simulink subsystem "Final_Project_PreBusUnpack_20260601_105527"  (R2024a)
settings: Solver=VariableStepAuto  StartTime=0.0  StopTime=10.0  RelTol=1e-3
values from neighbouring files (symbols this model uses):
  D = hypot(Ep(:,1)-Tp(:,1)',Ep(:,2)-Tp(:,2)')    [pp_compare_stage.m]    (also in pp_diag_path.m; pp_t09_clear.m = hypot(Ep(:,1)-Tperim(:,1)', Ep(:,2)-Tperim(:,2)'); pp_tune2.m)
undefined symbols (not defined in the file or in its folder): waypoints
libraries: CarMaker4SL x116, simulink x1
(part 1 of 7)
settings Model: Creator=junho.lee  LastModifiedBy=hajin

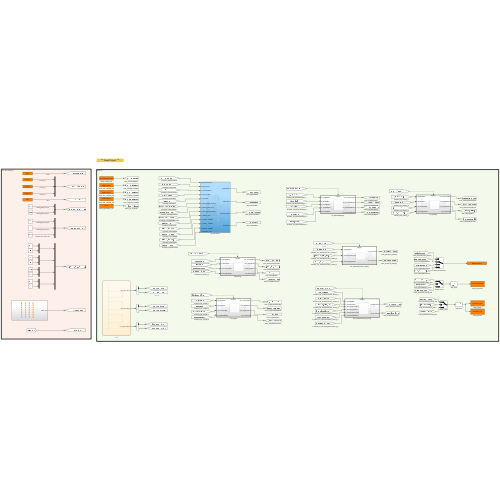
[thumbnail: Simulink's stored preview of the top-level diagram]
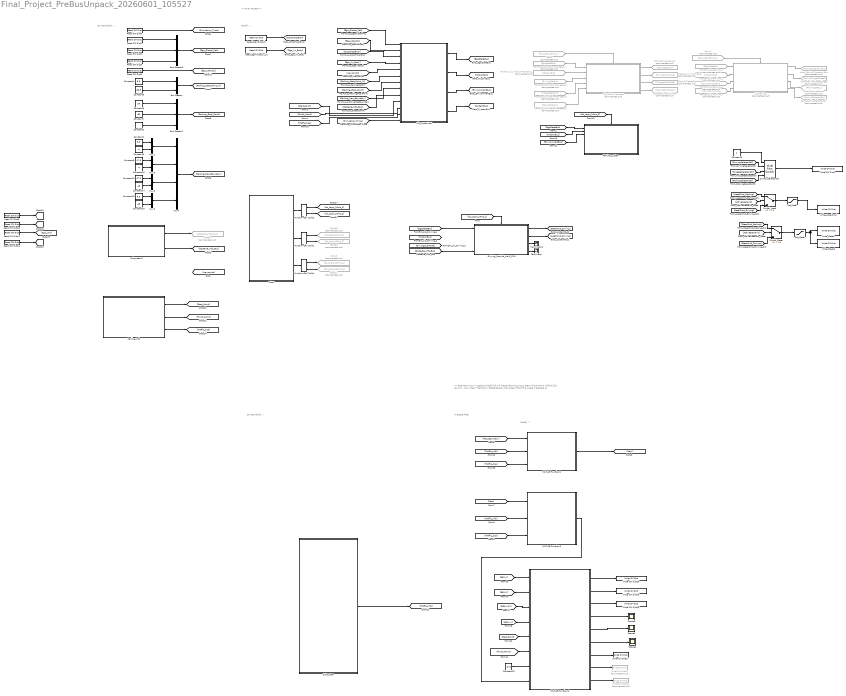
== system Final_Project_PreBusUnpack_20260601_105527 ==
  note: Do Not Modify !!
  note: *** Final Project ***
  note: Modify !!
  note: Do Not Modify !!
  note: Average Filter
  note: *** Path Planning ***
      |
      | Scenario: 장애물 회피 & 주차 Path Planning
      | Input: Start / Finish Point + 선행차량 정보 (Pos X/Y, Yaw, Size) + Collision / Object Sensor Info
      | Output: Front Tire Angle + Desired Ax
  note: Modify !!
  Bus Creator : BusCreator  Inputs=2
  Bus Creator1 : BusCreator  Inputs=3
  Bus Creator3 : BusCreator  Inputs=3
  Chart : Stateflow chart  TreatAsAtomicUnit=on
  Constant1 : Constant  Value=5.5
  Constant10 : Constant  Value=-4
  Constant13 : Constant  Value=47.5
  Constant14 : Constant  Value=-45
  Constant15 : Constant  Value=5.5
  Constant16 : Constant  Value=-45
  Constant2 : Constant  Value=2*pi/3
  Constant23 : Constant  Value=-pi/2
  Constant3 : Constant
  Constant4 : Constant  Value=5.5
  Constant5 : Constant  Value=-36.5
  Constant6 : Constant  Value=35
  Constant7 : Constant  Value=-30
  Constant8 : Constant  Value=47.5
  Constant9 : Constant  Value=-4
  Driving_Module_Ver.3_PSH : Subsystem
  From2 : From  Commented=on  GotoTag=do_Logic_50ms_1
  From5 : From  Commented=on  GotoTag=do_Logic_10ms_1
  FromExt_Lib_MissionManager_1 : From  Commented=on  GotoTag=EgoStateBus
  FromExt_Lib_MissionManager_2 : From  Commented=on  GotoTag=MissionBus
  FromExt_Lib_MissionManager_3 : From  Commented=on  GotoTag=DrivingStatus
  FromExt_Lib_MissionManager_4 : From  Commented=on  GotoTag=TollgateStatus
  FromExt_Lib_MissionManager_5 : From  Commented=on  GotoTag=ParkingStatus
  FromExt_Lib_Parking_1 : From  Commented=on  GotoTag=EgoStateBus
  FromExt_Lib_Parking_2 : From  Commented=on  GotoTag=MissionBus
  FromExt_Lib_Parking_3 : From  Commented=on  GotoTag=EnvironmentBus
  FromExt_Lib_Parking_4 : From  Commented=on  GotoTag=ParkingSubMode
  Function-Call Split1 : FunctionCallSplit  IconShape=distinctive  NumOutputPorts=2  OutputPortLayout=default
  Function-Call Split2 : FunctionCallSplit  IconShape=distinctive  NumOutputPorts=2  OutputPortLayout=default
  Function-Call Split4 : FunctionCallSplit  IconShape=distinctive  NumOutputPorts=2  OutputPortLayout=default
  Goto11 : Goto  Commented=on  GotoTag=do_Logic_100ms_2
  Goto28 : Goto  Commented=on  GotoTag=do_Logic_50ms_1
  Goto3 : Goto  Commented=on  GotoTag=do_Logic_100ms_1
  Goto30 : Goto  Commented=on  GotoTag=do_Logic_50ms_2
  Goto9 : Goto  Commented=on  GotoTag=Obstacle_Info_Mux
  Goto_ActiveScenario : Goto  Commented=on  GotoTag=ActiveScenario
  Goto_DrivingSubMode : Goto  Commented=on  GotoTag=DrivingSubMode
  Goto_ParkingSelectorCtrl : Goto  Commented=on  GotoTag=ParkingSelectorCtrl
  Goto_ParkingStatus : Goto  Commented=on  GotoTag=ParkingStatus
  Goto_ParkingSubMode : Goto  Commented=on  GotoTag=ParkingSubMode
  Goto_ParkingTargetSpeed : Goto  Commented=on  GotoTag=ParkingTargetSpeed
  Goto_ParkingTrajectoryBus : Goto  Commented=on  GotoTag=ParkingTrajectoryBus
  Goto_TollgateSubMode : Goto  Commented=on  GotoTag=TollgateSubMode
  Lib_MissionManager : Subsystem  Commented=on
  Lib_Parking : Subsystem  Commented=on
  Lib_Supervisor : Subsystem
  MATLAB Function2 : MATLAB Function  TreatAsAtomicUnit=on
  MATLAB Function3 : MATLAB Function  TreatAsAtomicUnit=on
  MATLAB Function6 : MATLAB Function  TreatAsAtomicUnit=on
  Mux{2,5,8..9} (4 alike) : Mux  Inputs=2
  Mux4 : Mux
  Parking_Info : Subsystem
  Parking_system : Subsystem
  Read CM Dict1 : CarMaker4SL/Read CM Dict  xname=Car.Fr1.tx  xsync=off  xstime=Inherited
  Read CM Dict10 : CarMaker4SL/Read CM Dict  xname=Car.Fr1.ty  xsync=off  xstime=Continuous
  Read CM Dict11 : CarMaker4SL/Read CM Dict  xname=Car.v  xsync=off  xstime=Continuous
  Read CM Dict12 : CarMaker4SL/Read CM Dict  xname=Car.Fr1.rz  xsync=off  xstime=Continuous
  Read CM Dict2 : CarMaker4SL/Read CM Dict  xname=Car.Fr1.ty  xsync=off  xstime=Inherited
  Read CM Dict3 : CarMaker4SL/Read CM Dict  xname=Car.Fr1.rz  xsync=off  xstime=Inherited
  Read CM Dict4 : CarMaker4SL/Read CM Dict  xname=Time  xsync=off  xstime=Inherited
  Read CM Dict5 : CarMaker4SL/Read CM Dict  xname=Car.v  xsync=off  xstime=Inherited
  Read CM Dict9 : CarMaker4SL/Read CM Dict  xname=Car.Fr1.tx  xsync=off  xstime=Continuous
  Read_DevDist_Lib : CarMaker4SL/Read CM Dict  xname=Car.Road.Path.DevDist  xsync=off  xstime=Inherited
  Read_EgoVxBody_Lib : CarMaker4SL/Read CM Dict  xname=Car.vx  xsync=off  xstime=Inherited
  Sat_Accel : Saturate  UpperLimit=3.0  LowerLimit=-5.0
  Sat_Steer : Saturate  UpperLimit=pi/6  LowerLimit=-pi/6
  Scope1 : Scope
  Scope2 : Scope
  Scope3 : Scope
  Subsystem : Subsystem
  Subsystem1 : Subsystem
  Switch_Accel : Switch  Criteria=u2 > Threshold  Threshold=2.5
  Switch_SelectorCtrl : MultiPortSwitch  DataPortOrder=Specify indices  DataPortIndices={1, 2, 3}  OutDataTypeStr=double
  Switch_Steer : Switch  Criteria=u2 > Threshold  Threshold=2.5
  Terminator : Terminator
  Terminator1 : Terminator
  Write CM Dict14 : CarMaker4SL/Write CM Dict  xname=Car.CFL.rz_ext  xsync=off
  Write CM Dict15 : CarMaker4SL/Write CM Dict  xname=Car.CFR.rz_ext  xsync=off
  Write CM Dict16 : CarMaker4SL/Write CM Dict  Commented=on  xname=VC.Brake  xsync=off
  Write CM Dict17 : CarMaker4SL/Write CM Dict  xname=DM.SelectorCtrl  xsync=off
  Write CM Dict18 : CarMaker4SL/Write CM Dict  Commented=on  xname=VC.Gas  xsync=off
  Write CM Dict19 : CarMaker4SL/Write CM Dict  xname=AccelCtrl.DesiredAx  xsync=off
  Write CM Dict4 : CarMaker4SL/Write CM Dict  xname=DM.SelectorCtrl  xsync=off
  Write_AccelCmd : CarMaker4SL/Write CM Dict  xname=AccelCtrl.DesiredAx  xsync=off
  Write_SteerL : CarMaker4SL/Write CM Dict  xname=Car.CFL.rz_ext  xsync=off
  Write_SteerR : CarMaker4SL/Write CM Dict  xname=Car.CFR.rz_ext  xsync=off
  wires:
  Constant13/1 -> Mux8/1
  Subsystem1/1(Traffic_Info) -> Goto9/1
  Read CM Dict1/1 -> Bus Creator3/1  "Car_Fr1_tx"
  Read CM Dict3/1 -> Bus Creator3/3  "Car_Fr1_rz"
  Constant4/1 -> Bus Creator/1  "Parking_Start_Point_X"
  Chart/2(do_Logic_50ms()) -> Function-Call Split1/1
  Function-Call Split2/1 -> [do_Logic_10ms_1]
  Function-Call Split1/2 -> Goto30/1
  Read CM Dict4/1 -> [Simulation_Time]  "Time"
  Constant9/1 -> Mux2/2
  Bus Creator1/1 -> [Parking_Goal_Point]
  Mux8/1 -> Mux4/3
  Constant6/1 -> Bus Creator1/1  "Parking_Goal_Point_X"
  Constant1/1 -> Mux2/1
  Constant16/1 -> Mux9/2
  Read CM Dict2/1 -> Bus Creator3/2  "Car_Fr1_ty"
  Function-Call Split1/1 -> Goto28/1
  Constant5/1 -> Bus Creator/2  "Parking_Start_Point_Y"
  Chart/1(do_Logic_10ms()) -> Function-Call Split2/1
  Constant7/1 -> Bus Creator1/2  "Parking_Goal_Point_Y"
  Read CM Dict5/1 -> [Ego_Velocity]  "Car.v"
  Constant15/1 -> Mux9/1
  Constant10/1 -> Mux5/2
  Bus Creator3/1 -> [Ego_Global_Pos]
  Constant14/1 -> Mux8/2
  Function-Call Split2/2 -> [do_Logic_10ms_2]
  Bus Creator/1 -> [Parking_Start_Point_XY]
  Mux9/1 -> Mux4/4
  Mux2/1 -> Mux4/1
  Mux4/1 -> [Parking_Map_Boundary]
  Constant8/1 -> Mux5/1
  Constant2/1 -> Bus Creator1/3  "Parking_Goal_Point_Yaw"
  Mux5/1 -> Mux4/2
  Chart/3(do_Logic_100ms()) -> Function-Call Split4/1
  Function-Call Split4/1 -> Goto3/1
  Function-Call Split4/2 -> Goto11/1
  Sat_Steer/1 -> Write_SteerR/1, Write_SteerL/1
  Read_DevDist_Lib/1 -> [CrossTrackError]
  Read_EgoVxBody_Lib/1 -> [Ego_Vx_Body]
  [Ego_Global_Pos] -> Lib_Supervisor/1(In_Ego_Global_Pos)
  [Ego_Velocity] -> Lib_Supervisor/2(In_Ego_Velocity)
  [CrossTrackError] -> Lib_Supervisor/3(In_CrossTrackError)
  [Ego_Vx_Body] -> Lib_Supervisor/4(In_Ego_Vx_Body)
  [waypoints] -> Lib_Supervisor/5(In_Waypoints)
  [Parking_Start_Point_XY] -> Lib_Supervisor/6(In_Parking_Start_Point_XY)
  [Parking_Goal_Point] -> Lib_Supervisor/7(In_Parking_Goal_Point)
  [Parking_Map_Boundary] -> Lib_Supervisor/8(In_Parking_Map_Boundary)
  [Simulation_Time] -> Lib_Supervisor/13(In_Simulation_Time)
  Lib_Supervisor/1(EgoStateBus) -> [EgoStateBus]
  Lib_Supervisor/2(MissionBus) -> [MissionBus]
  Lib_Supervisor/3(EnvironmentBus) -> [EnvironmentBus]
  Lib_Supervisor/4(SystemBus) -> [SystemBus]
  Lib_MissionManager/1(Out_ActiveScenario) -> Goto_ActiveScenario/1
  Lib_MissionManager/2(Out_DrivingSubMode) -> Goto_DrivingSubMode/1
  Lib_MissionManager/3(Out_TollgateSubMode) -> Goto_TollgateSubMode/1
  Lib_MissionManager/4(Out_ParkingSubMode) -> Goto_ParkingSubMode/1
  Lib_Parking/1(Out_TrajectoryBus) -> Goto_ParkingTrajectoryBus/1
  Lib_Parking/2(Out_TargetSpeed) -> Goto_ParkingTargetSpeed/1
  Lib_Parking/3(Out_ParkingStatus) -> Goto_ParkingStatus/1
  FromExt_Lib_MissionManager_1/1 -> Lib_MissionManager/1(In_EgoStateBus)
  FromExt_Lib_MissionManager_2/1 -> Lib_MissionManager/2(In_MissionBus)
  FromExt_Lib_MissionManager_3/1 -> Lib_MissionManager/3(In_DrivingStatus)
  FromExt_Lib_MissionManager_4/1 -> Lib_MissionManager/4(In_TollgateStatus)
  FromExt_Lib_MissionManager_5/1 -> Lib_MissionManager/5(In_ParkingStatus)
  [EgoStateBus] -> Driving_Module_Ver.3_PSH/1(In_EgoStateBus)
  FromExt_Lib_Parking_1/1 -> Lib_Parking/1(In_EgoStateBus)
  FromExt_Lib_Parking_2/1 -> Lib_Parking/2(In_MissionBus)
  FromExt_Lib_Parking_3/1 -> Lib_Parking/3(In_EnvironmentBus)
  FromExt_Lib_Parking_4/1 -> Lib_Parking/4(In_ParkingSubMode)
  From5/1 -> Lib_MissionManager/Trigger
  [do_Logic_10ms_1] -> Driving_Module_Ver.3_PSH/Trigger
  From2/1 -> Lib_Parking/Trigger
  [SteerCmd_Parking] -> Switch_Steer/1
  [ActiveScenario] -> Switch_Steer/2
  [SteerCmd_Driving] -> Switch_Steer/3
  Switch_Steer/1 -> Sat_Steer/1
  [AccelCmd_Parking] -> Switch_Accel/1
  [ActiveScenario] -> Switch_Accel/2
  [AccelCmd_Driving] -> Switch_Accel/3
  Switch_Accel/1 -> Sat_Accel/1
  Lib_Parking/4(Out_SelectorCtrl) -> Goto_ParkingSelectorCtrl/1
  [DrivingSelectorCtrl] -> Switch_SelectorCtrl/2
  [TollgateSelectorCtrl] -> Switch_SelectorCtrl/3
  [ParkingSelectorCtrl] -> Switch_SelectorCtrl/4
  Switch_SelectorCtrl/1 -> Write CM Dict4/1
  Constant3/1 -> Switch_SelectorCtrl/1
  Sat_Accel/1 -> Write_AccelCmd/1
  Subsystem1/2(Outport) -> [Obstacle_Info_Bus]
  [Obstacle_Info_Bus] -> Lib_Supervisor/9(In_Obstacle_Info)
  Driving_Module_Ver.3_PSH/1(SteerCmd_Driving) -> [SteerCmd_Driving]
  Driving_Module_Ver.3_PSH/2(AccelCmd_Driving) -> [AccelCmd_Driving]
  [Obstacle_Info_Bus] -> Driving_Module_Ver.3_PSH/4(Obstacle_Info_Bus)
  Driving_Module_Ver.3_PSH/4(mission_state) -> Terminator/1
  Driving_Module_Ver.3_PSH/3(Gear_Pos) -> Terminator1/1
  [ego_y] -> MATLAB Function6/2(ego_y)
  [Start_Point] -> MATLAB Function6/5(start_point)
  MATLAB Function6/5(path_y_dbg) -> Scope2/1
  MATLAB Function6/7(selector_ctrl) -> Write CM Dict17/1
  MATLAB Function6/1(desired_ax) -> Write CM Dict19/1
  [ego_yaw] -> MATLAB Function6/3(ego_yaw)
  [Traffic_size] -> MATLAB Function2/3(traffic_size)
  [Traffic_Info] -> MATLAB Function2/2(traffic_info)
  MATLAB Function6/8(vc_gas) -> Write CM Dict18/1
  Subsystem/1(Traffic_Info) -> [Traffic_Info]
  [ego_x] -> MATLAB Function6/1(ego_x)
  MATLAB Function6/4(path_x_dbg) -> Scope3/1
  [Traffic_size] -> MATLAB Function3/3(traffic_size)
  [Map] -> MATLAB Function3/1(map)
  MATLAB Function6/9(vc_brake) -> Write CM Dict16/1
  MATLAB Function6/3(steer_fr) -> Write CM Dict15/1
  MATLAB Function6/2(steer_fl) -> Write CM Dict14/1
  Constant23/1 -> MATLAB Function6/7(goal_yaw)
  [Traffic_Info] -> MATLAB Function3/2(traffic_info)
  MATLAB Function6/6(path_len_dbg) -> Scope1/1
  [ego_vx] -> MATLAB Function6/4(ego_v)
  [Finish_Point] -> MATLAB Function6/6(finish_point)
  MATLAB Function3/1(y) -> MATLAB Function6/8(occ_map)
  MATLAB Function2/1(mapMatrix) -> [Map]
  [Map_Boundary] -> MATLAB Function2/1(map_boundary)
  Read CM Dict12/1 -> [ego_yaw]
  Read CM Dict11/1 -> [ego_vx]
  Read CM Dict9/1 -> [ego_x]
  Read CM Dict10/1 -> [ego_y]
  Parking_Info/1(Start_Point) -> [Start_Point]
  Parking_Info/2(Finish_Point) -> [Finish_Point]
  Parking_Info/3(Traffic_size) -> [Traffic_size]
  [Start_Point] -> Lib_Supervisor/10(Start_Point)
  [Finish_Point] -> Lib_Supervisor/11(Finish_Point)
  [Traffic_size] -> Lib_Supervisor/12(Traffic_size)
  [do_Logic_10ms_2] -> Parking_system/Trigger
  [EgoStateBus] -> Parking_system/1(In_EgoStateBus)
  [EnvironmentBus] -> Parking_system/3(In_EnvironmentBus)
  [MissionBus] -> Parking_system/2(In_MissionBus)

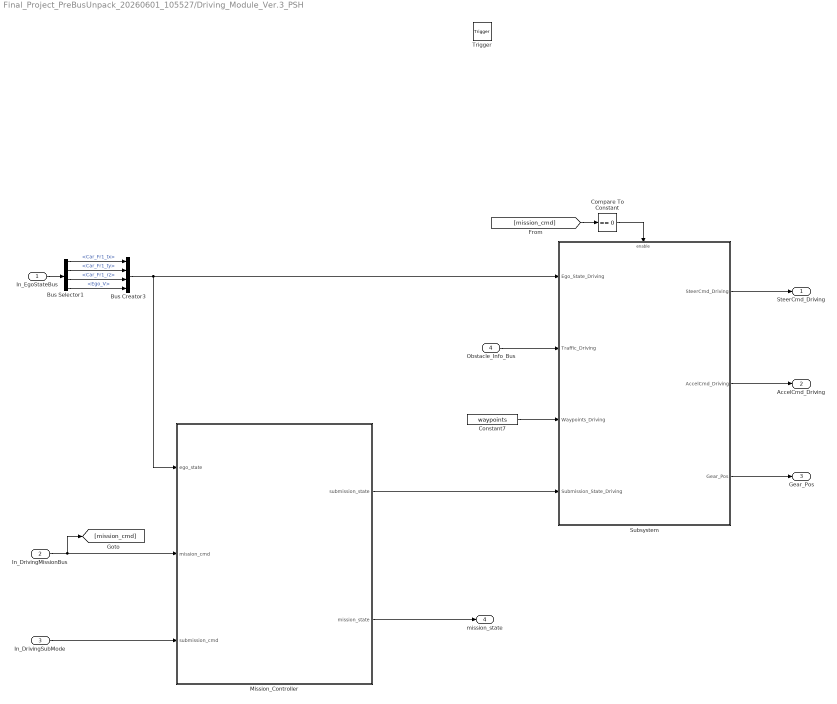
== system Final_Project_PreBusUnpack_20260601_105527/Driving_Module_Ver.3_PSH ==
  In_EgoStateBus : Inport
  In_DrivingMissionBus : Inport  Port=2
  In_DrivingSubMode : Inport  Port=3
  Obstacle_Info_Bus : Inport  Port=4
  Trigger : TriggerPort  TriggerType=function-call  VariantControl=(inherit)
  Bus Creator3 : BusCreator  Inputs=4  OutDataTypeStr=Bus: EgoStateBus
  Bus Selector1 : BusSelector  OutputSignals=Car_Fr1_tx,Car_Fr1_ty,Car_Fr1_rz,Ego_V
  Compare To Constant : simulink/Logic and Bit Operations/Compare To Constant  relop===  const=0  OutDataTypeStr=boolean
  Constant7 : Constant  Value=waypoints
  Mission_Controller : MATLAB Function  TreatAsAtomicUnit=on
  Subsystem : Subsystem
  SteerCmd_Driving : Outport
  AccelCmd_Driving : Outport  Port=2
  Gear_Pos : Outport  Port=3
  mission_state : Outport  Port=4
  wires:
  Subsystem/3(Gear_Pos) -> Gear_Pos/1
  Compare To Constant/1 -> Subsystem/Enable
  [mission_cmd] -> Compare To Constant/1
  In_DrivingMissionBus/1 -> [mission_cmd], Mission_Controller/2(mission_cmd)
  In_DrivingSubMode/1 -> Mission_Controller/3(submission_cmd)
  Mission_Controller/2(mission_state) -> mission_state/1
  In_EgoStateBus/1 -> Bus Selector1/1
  Bus Selector1/4 -> Bus Creator3/4  "<Ego_V>"
  Bus Creator3/1 -> Mission_Controller/1(ego_state), Subsystem/1(Ego_State_Driving)
  Bus Selector1/3 -> Bus Creator3/3  "<Car_Fr1_rz>"
  Bus Selector1/2 -> Bus Creator3/2  "<Car_Fr1_ty>"
  Bus Selector1/1 -> Bus Creator3/1  "<Car_Fr1_tx>"
  Mission_Controller/1(submission_state) -> Subsystem/4(Submission_State_Driving)
  Constant7/1 -> Subsystem/3(Waypoints_Driving)
  Obstacle_Info_Bus/1 -> Subsystem/2(Traffic_Driving)
  Subsystem/2(AccelCmd_Driving) -> AccelCmd_Driving/1
  Subsystem/1(SteerCmd_Driving) -> SteerCmd_Driving/1

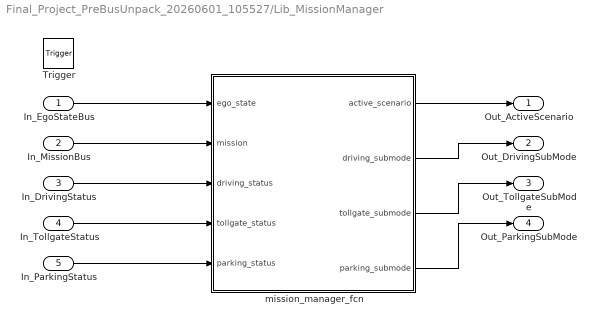
== system Final_Project_PreBusUnpack_20260601_105527/Lib_MissionManager ==
  In_EgoStateBus : Inport
  In_MissionBus : Inport  Port=2
  In_DrivingStatus : Inport  Port=3
  In_TollgateStatus : Inport  Port=4
  In_ParkingStatus : Inport  Port=5
  Trigger : TriggerPort  TriggerType=function-call  VariantControl=(inherit)
  mission_manager_fcn : MATLAB Function  TreatAsAtomicUnit=on
  Out_ActiveScenario : Outport
  Out_DrivingSubMode : Outport  Port=2
  Out_TollgateSubMode : Outport  Port=3
  Out_ParkingSubMode : Outport  Port=4
  wires:
  In_EgoStateBus/1 -> mission_manager_fcn/1(ego_state)
  In_MissionBus/1 -> mission_manager_fcn/2(mission)
  In_DrivingStatus/1 -> mission_manager_fcn/3(driving_status)
  In_TollgateStatus/1 -> mission_manager_fcn/4(tollgate_status)
  In_ParkingStatus/1 -> mission_manager_fcn/5(parking_status)
  mission_manager_fcn/1(active_scenario) -> Out_ActiveScenario/1
  mission_manager_fcn/2(driving_submode) -> Out_DrivingSubMode/1
  mission_manager_fcn/3(tollgate_submode) -> Out_TollgateSubMode/1
  mission_manager_fcn/4(parking_submode) -> Out_ParkingSubMode/1

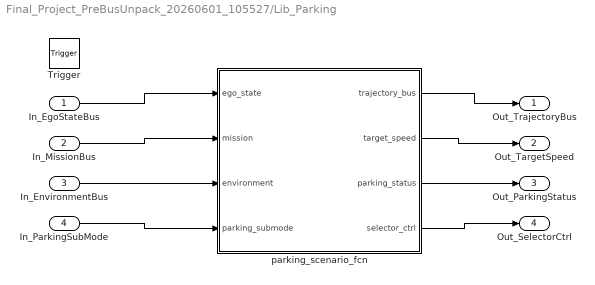
== system Final_Project_PreBusUnpack_20260601_105527/Lib_Parking ==
  In_EgoStateBus : Inport
  In_MissionBus : Inport  Port=2
  In_EnvironmentBus : Inport  Port=3
  In_ParkingSubMode : Inport  Port=4
  Trigger : TriggerPort  TriggerType=function-call  VariantControl=(inherit)
  parking_scenario_fcn : MATLAB Function  TreatAsAtomicUnit=on
  Out_TrajectoryBus : Outport
  Out_TargetSpeed : Outport  Port=2
  Out_ParkingStatus : Outport  Port=3
  Out_SelectorCtrl : Outport  Port=4
  wires:
  In_EgoStateBus/1 -> parking_scenario_fcn/1(ego_state)
  In_MissionBus/1 -> parking_scenario_fcn/2(mission)
  In_EnvironmentBus/1 -> parking_scenario_fcn/3(environment)
  In_ParkingSubMode/1 -> parking_scenario_fcn/4(parking_submode)
  parking_scenario_fcn/1(trajectory_bus) -> Out_TrajectoryBus/1
  parking_scenario_fcn/2(target_speed) -> Out_TargetSpeed/1
  parking_scenario_fcn/3(parking_status) -> Out_ParkingStatus/1
  parking_scenario_fcn/4(selector_ctrl) -> Out_SelectorCtrl/1

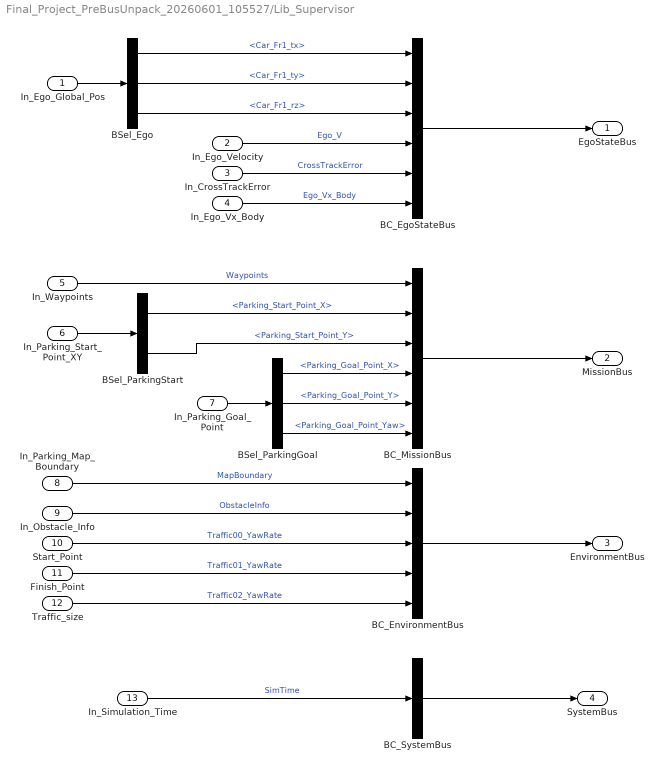
== system Final_Project_PreBusUnpack_20260601_105527/Lib_Supervisor ==
  In_Ego_Global_Pos : Inport
  In_Ego_Velocity : Inport  Port=2
  In_CrossTrackError : Inport  Port=3
  In_Ego_Vx_Body : Inport  Port=4
  In_Waypoints : Inport  Port=5
  In_Parking_Start_Point_XY : Inport  Port=6
  In_Parking_Goal_Point : Inport  Port=7
  In_Parking_Map_Boundary : Inport  Port=8
  In_Obstacle_Info : Inport  Port=9
  Start_Point : Inport  Port=10
  Finish_Point : Inport  Port=11
  Traffic_size : Inport  Port=12
  In_Simulation_Time : Inport  Port=13
  BC_EgoStateBus : BusCreator  Inputs=6
  BC_EnvironmentBus : BusCreator  Inputs=5
  BC_MissionBus : BusCreator  Inputs=6
  BC_SystemBus : BusCreator  Inputs=1
  BSel_Ego : BusSelector  OutputSignals=Car_Fr1_tx,Car_Fr1_ty,Car_Fr1_rz
  BSel_ParkingGoal : BusSelector  OutputSignals=Parking_Goal_Point_X,Parking_Goal_Point_Y,Parking_Goal_Point_Yaw
  BSel_ParkingStart : BusSelector  OutputSignals=Parking_Start_Point_X,Parking_Start_Point_Y
  EgoStateBus : Outport
  MissionBus : Outport  Port=2
  EnvironmentBus : Outport  Port=3
  SystemBus : Outport  Port=4
  wires:
  In_Ego_Global_Pos/1 -> BSel_Ego/1
  In_Parking_Start_Point_XY/1 -> BSel_ParkingStart/1
  In_Parking_Goal_Point/1 -> BSel_ParkingGoal/1
  BSel_Ego/1 -> BC_EgoStateBus/1  "<Car_Fr1_tx>"
  BSel_Ego/2 -> BC_EgoStateBus/2  "<Car_Fr1_ty>"
  BSel_Ego/3 -> BC_EgoStateBus/3  "<Car_Fr1_rz>"
  In_Ego_Velocity/1 -> BC_EgoStateBus/4  "Ego_V"
  In_CrossTrackError/1 -> BC_EgoStateBus/5  "CrossTrackError"
  In_Ego_Vx_Body/1 -> BC_EgoStateBus/6  "Ego_Vx_Body"
  In_Waypoints/1 -> BC_MissionBus/1  "Waypoints"
  BSel_ParkingStart/1 -> BC_MissionBus/2  "<Parking_Start_Point_X>"
  BSel_ParkingStart/2 -> BC_MissionBus/3  "<Parking_Start_Point_Y>"
  BSel_ParkingGoal/1 -> BC_MissionBus/4  "<Parking_Goal_Point_X>"
  BSel_ParkingGoal/2 -> BC_MissionBus/5  "<Parking_Goal_Point_Y>"
  BSel_ParkingGoal/3 -> BC_MissionBus/6  "<Parking_Goal_Point_Yaw>"
  In_Parking_Map_Boundary/1 -> BC_EnvironmentBus/1  "MapBoundary"
  In_Obstacle_Info/1 -> BC_EnvironmentBus/2  "ObstacleInfo"
  Start_Point/1 -> BC_EnvironmentBus/3  "Traffic00_YawRate"
  Finish_Point/1 -> BC_EnvironmentBus/4  "Traffic01_YawRate"
  Traffic_size/1 -> BC_EnvironmentBus/5  "Traffic02_YawRate"
  In_Simulation_Time/1 -> BC_SystemBus/1  "SimTime"
  BC_EgoStateBus/1 -> EgoStateBus/1
  BC_MissionBus/1 -> MissionBus/1
  BC_EnvironmentBus/1 -> EnvironmentBus/1
  BC_SystemBus/1 -> SystemBus/1

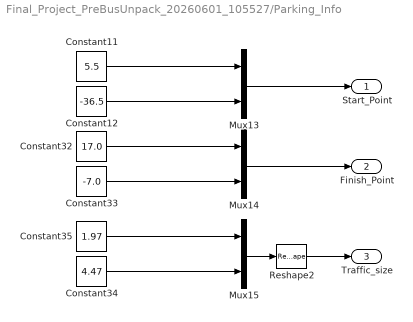
== system Final_Project_PreBusUnpack_20260601_105527/Parking_Info ==
  Constant11 : Constant  Value=5.5
  Constant12 : Constant  Value=-36.5
  Constant32 : Constant  Value=17.0
  Constant33 : Constant  Value=-7.0
  Constant34 : Constant  Value=4.47
  Constant35 : Constant  Value=1.97
  Mux13 : Mux  Inputs=2
  Mux14 : Mux  Inputs=2
  Mux15 : Mux  Inputs=2
  Reshape2 : Reshape  OutputDimensionality=Row vector (2-D)  OutputDimensions=[2,2]
  Start_Point : Outport
  Finish_Point : Outport  Port=2
  Traffic_size : Outport  Port=3
  wires:
  Constant12/1 -> Mux13/2
  Constant11/1 -> Mux13/1
  Constant33/1 -> Mux14/2
  Mux13/1 -> Start_Point/1
  Reshape2/1 -> Traffic_size/1
  Mux15/1 -> Reshape2/1
  Constant32/1 -> Mux14/1
  Constant34/1 -> Mux15/2
  Constant35/1 -> Mux15/1
  Mux14/1 -> Finish_Point/1

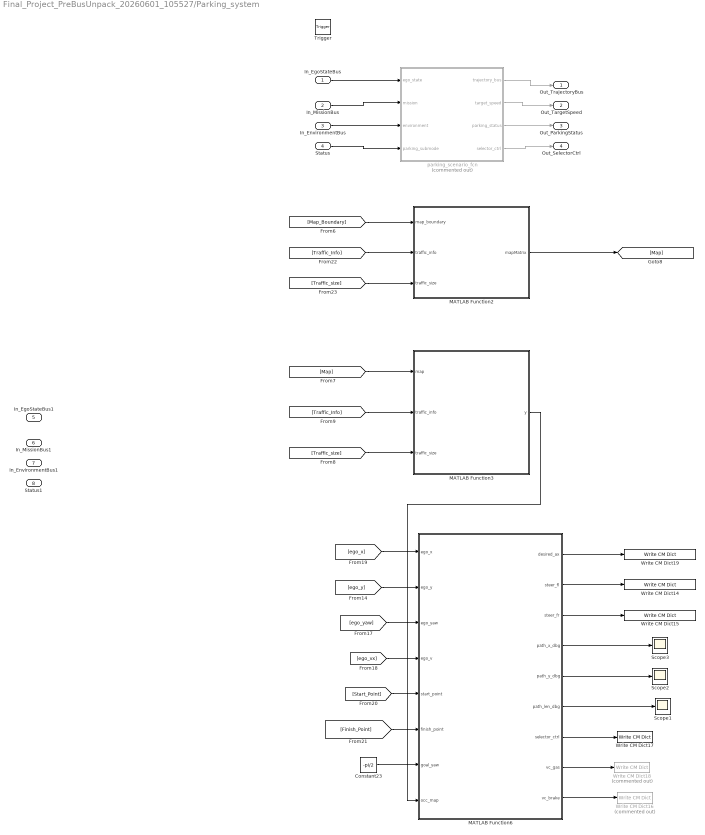
== system Final_Project_PreBusUnpack_20260601_105527/Parking_system ==
  In_EgoStateBus : Inport
  In_MissionBus : Inport  Port=2
  In_EnvironmentBus : Inport  Port=3
  Status : Inport  Port=4
  In_EgoStateBus1 : Inport  Port=5
  In_MissionBus1 : Inport  Port=6
  In_EnvironmentBus1 : Inport  Port=7
  Status1 : Inport  Port=8
  Trigger : TriggerPort  TriggerType=function-call  VariantControl=(inherit)
  Constant23 : Constant  Value=-pi/2
  MATLAB Function2 : MATLAB Function  TreatAsAtomicUnit=on
  MATLAB Function3 : MATLAB Function  TreatAsAtomicUnit=on
  MATLAB Function6 : MATLAB Function  TreatAsAtomicUnit=on
  Scope1 : Scope
  Scope2 : Scope
  Scope3 : Scope
  Write CM Dict14 : CarMaker4SL/Write CM Dict  xname=Car.CFL.rz_ext  xsync=off
  Write CM Dict15 : CarMaker4SL/Write CM Dict  xname=Car.CFR.rz_ext  xsync=off
  Write CM Dict16 : CarMaker4SL/Write CM Dict  Commented=on  xname=VC.Brake  xsync=off
  Write CM Dict17 : CarMaker4SL/Write CM Dict  xname=DM.SelectorCtrl  xsync=off
  Write CM Dict18 : CarMaker4SL/Write CM Dict  Commented=on  xname=VC.Gas  xsync=off
  Write CM Dict19 : CarMaker4SL/Write CM Dict  xname=AccelCtrl.DesiredAx  xsync=off
  parking_scenario_fcn : MATLAB Function  Commented=on  TreatAsAtomicUnit=on
  Out_TrajectoryBus : Outport
  Out_TargetSpeed : Outport  Port=2
  Out_ParkingStatus : Outport  Port=3
  Out_SelectorCtrl : Outport  Port=4
  wires:
  MATLAB Function6/9(vc_brake) -> Write CM Dict16/1
  MATLAB Function6/8(vc_gas) -> Write CM Dict18/1
  MATLAB Function6/7(selector_ctrl) -> Write CM Dict17/1
  MATLAB Function6/6(path_len_dbg) -> Scope1/1
  MATLAB Function6/5(path_y_dbg) -> Scope2/1
  MATLAB Function6/4(path_x_dbg) -> Scope3/1
  MATLAB Function6/3(steer_fr) -> Write CM Dict15/1
  MATLAB Function6/2(steer_fl) -> Write CM Dict14/1
  MATLAB Function6/1(desired_ax) -> Write CM Dict19/1
  MATLAB Function3/1(y) -> MATLAB Function6/8(occ_map)
  Constant23/1 -> MATLAB Function6/7(goal_yaw)
  [Finish_Point] -> MATLAB Function6/6(finish_point)
  [Start_Point] -> MATLAB Function6/5(start_point)
  [ego_vx] -> MATLAB Function6/4(ego_v)
  [ego_yaw] -> MATLAB Function6/3(ego_yaw)
  [ego_y] -> MATLAB Function6/2(ego_y)
  [ego_x] -> MATLAB Function6/1(ego_x)
  [Traffic_size] -> MATLAB Function3/3(traffic_size)
  [Traffic_Info] -> MATLAB Function3/2(traffic_info)
  [Map] -> MATLAB Function3/1(map)
  MATLAB Function2/1(mapMatrix) -> [Map]
  [Traffic_size] -> MATLAB Function2/3(traffic_size)
  [Traffic_Info] -> MATLAB Function2/2(traffic_info)
  [Map_Boundary] -> MATLAB Function2/1(map_boundary)
  In_EgoStateBus/1 -> parking_scenario_fcn/1(ego_state)
  In_MissionBus/1 -> parking_scenario_fcn/2(mission)
  In_EnvironmentBus/1 -> parking_scenario_fcn/3(environment)
  Status/1 -> parking_scenario_fcn/4(parking_submode)
  parking_scenario_fcn/1(trajectory_bus) -> Out_TrajectoryBus/1
  parking_scenario_fcn/2(target_speed) -> Out_TargetSpeed/1
  parking_scenario_fcn/3(parking_status) -> Out_ParkingStatus/1
  parking_scenario_fcn/4(selector_ctrl) -> Out_SelectorCtrl/1

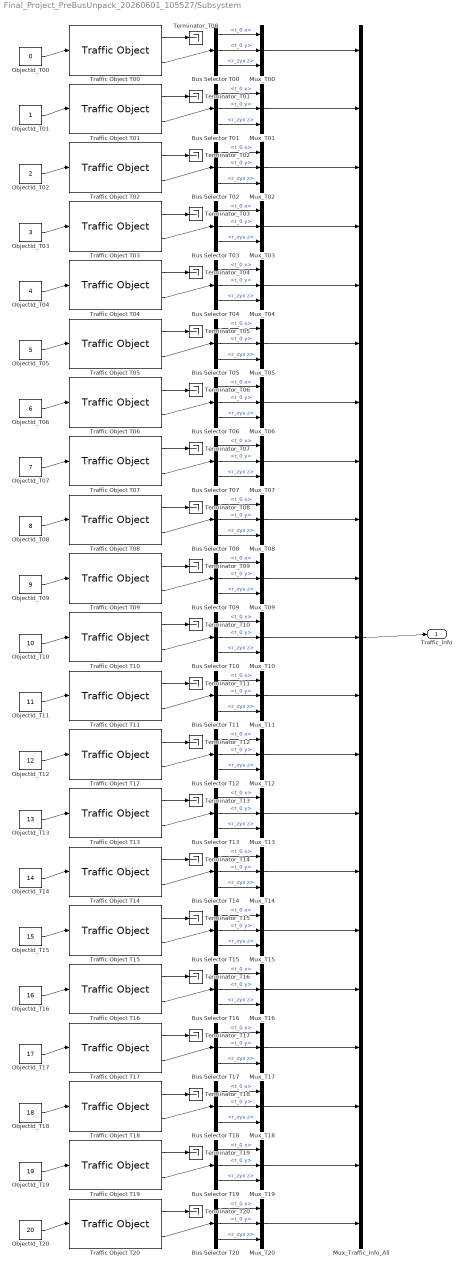
== system Final_Project_PreBusUnpack_20260601_105527/Subsystem ==
  Bus Selector T00 : BusSelector  OutputSignals=t_0 x,t_0 y,r_zyx z
  Bus Selector T01 : BusSelector  OutputSignals=t_0 x,t_0 y,r_zyx z
  Bus Selector T02 : BusSelector  OutputSignals=t_0 x,t_0 y,r_zyx z
  Bus Selector T03 : BusSelector  OutputSignals=t_0 x,t_0 y,r_zyx z
  Bus Selector T04 : BusSelector  OutputSignals=t_0 x,t_0 y,r_zyx z
  Bus Selector T05 : BusSelector  OutputSignals=t_0 x,t_0 y,r_zyx z
  Bus Selector T06 : BusSelector  OutputSignals=t_0 x,t_0 y,r_zyx z
  Bus Selector T07 : BusSelector  OutputSignals=t_0 x,t_0 y,r_zyx z
  Bus Selector T08 : BusSelector  OutputSignals=t_0 x,t_0 y,r_zyx z
  Bus Selector T09 : BusSelector  OutputSignals=t_0 x,t_0 y,r_zyx z
  Bus Selector T{10..20} (11 alike) : BusSelector  OutputSignals=t_0 x,t_0 y,r_zyx z
  Mux_T00 : Mux  Inputs=3
  Mux_T01 : Mux  Inputs=3
  Mux_T02 : Mux  Inputs=3
  Mux_T03 : Mux  Inputs=3
  Mux_T04 : Mux  Inputs=3
  Mux_T05 : Mux  Inputs=3
  Mux_T06 : Mux  Inputs=3
  Mux_T07 : Mux  Inputs=3
  Mux_T08 : Mux  Inputs=3
  Mux_T09 : Mux  Inputs=3
  Mux_T{10..20} (11 alike) : Mux  Inputs=3
  Mux_Traffic_Info_All : Mux  Inputs=21
  ObjectId_T00 : Constant  Value=0
  ObjectId_T01 : Constant
  ObjectId_T02 : Constant  Value=2
  ObjectId_T03 : Constant  Value=3
  ObjectId_T04 : Constant  Value=4
  ObjectId_T05 : Constant  Value=5
  ObjectId_T06 : Constant  Value=6
  ObjectId_T07 : Constant  Value=7
  ObjectId_T08 : Constant  Value=8
  ObjectId_T09 : Constant  Value=9
  ObjectId_T10 : Constant  Value=10
  ObjectId_T11 : Constant  Value=11
  ObjectId_T12 : Constant  Value=12
  ObjectId_T13 : Constant  Value=13
  ObjectId_T14 : Constant  Value=14
  ObjectId_T15 : Constant  Value=15
  ObjectId_T16 : Constant  Value=16
  ObjectId_T17 : Constant  Value=17
  ObjectId_T18 : Constant  Value=18
  ObjectId_T19 : Constant  Value=19
  ObjectId_T20 : Constant  Value=20
  Terminator_T00 : Terminator
  Terminator_T01 : Terminator
  Terminator_T02 : Terminator
  Terminator_T03 : Terminator
  Terminator_T04 : Terminator
  Terminator_T05 : Terminator
  Terminator_T06 : Terminator
  Terminator_T07 : Terminator
  Terminator_T08 : Terminator
  Terminator_T09 : Terminator
  Terminator_T{10..20} (11 alike) : Terminator
  Traffic Object T00 : CarMaker4SL/Traffic Object  xname=T00  ximode=Traffic Id  xstime=Inherited
      settings: SourceProductName=CarMaker4SL
  Traffic Object T01 : CarMaker4SL/Traffic Object  xname=T01  ximode=Traffic Id  xstime=Inherited
      settings: SourceProductName=CarMaker4SL
  Traffic Object T02 : CarMaker4SL/Traffic Object  xname=T02  ximode=Traffic Id  xstime=Inherited
      settings: SourceProductName=CarMaker4SL
  Traffic Object T03 : CarMaker4SL/Traffic Object  xname=T03  ximode=Traffic Id  xstime=Inherited
      settings: SourceProductName=CarMaker4SL
  Traffic Object T04 : CarMaker4SL/Traffic Object  xname=T04  ximode=Traffic Id  xstime=Inherited
      settings: SourceProductName=CarMaker4SL
  Traffic Object T05 : CarMaker4SL/Traffic Object  xname=T05  ximode=Traffic Id  xstime=Inherited
      settings: SourceProductName=CarMaker4SL
  Traffic Object T06 : CarMaker4SL/Traffic Object  xname=T06  ximode=Traffic Id  xstime=Inherited
      settings: SourceProductName=CarMaker4SL
  Traffic Object T07 : CarMaker4SL/Traffic Object  xname=T07  ximode=Traffic Id  xstime=Inherited
      settings: SourceProductName=CarMaker4SL
  Traffic Object T08 : CarMaker4SL/Traffic Object  xname=T08  ximode=Traffic Id  xstime=Inherited
      settings: SourceProductName=CarMaker4SL
  Traffic Object T09 : CarMaker4SL/Traffic Object  xname=T09  ximode=Traffic Id  xstime=Inherited
      settings: SourceProductName=CarMaker4SL
  Traffic Object T10 : CarMaker4SL/Traffic Object  xname=T10  ximode=Traffic Id  xstime=Inherited
      settings: SourceProductName=CarMaker4SL
  Traffic Object T11 : CarMaker4SL/Traffic Object  xname=T11  ximode=Traffic Id  xstime=Inherited
      settings: SourceProductName=CarMaker4SL
  Traffic Object T12 : CarMaker4SL/Traffic Object  xname=T12  ximode=Traffic Id  xstime=Inherited
      settings: SourceProductName=CarMaker4SL
  Traffic Object T13 : CarMaker4SL/Traffic Object  xname=T13  ximode=Traffic Id  xstime=Inherited
      settings: SourceProductName=CarMaker4SL
  Traffic Object T14 : CarMaker4SL/Traffic Object  xname=T14  ximode=Traffic Id  xstime=Inherited
      settings: SourceProductName=CarMaker4SL
  Traffic Object T15 : CarMaker4SL/Traffic Object  xname=T15  ximode=Traffic Id  xstime=Inherited
      settings: SourceProductName=CarMaker4SL
  Traffic Object T16 : CarMaker4SL/Traffic Object  xname=T16  ximode=Traffic Id  xstime=Inherited
      settings: SourceProductName=CarMaker4SL
  Traffic Object T17 : CarMaker4SL/Traffic Object  xname=T17  ximode=Traffic Id  xstime=Inherited
      settings: SourceProductName=CarMaker4SL
  Traffic Object T18 : CarMaker4SL/Traffic Object  xname=T18  ximode=Traffic Id  xstime=Inherited
      settings: SourceProductName=CarMaker4SL
  Traffic Object T19 : CarMaker4SL/Traffic Object  xname=T19  ximode=Traffic Id  xstime=Inherited
      settings: SourceProductName=CarMaker4SL
  Traffic Object T20 : CarMaker4SL/Traffic Object  xname=T20  ximode=Traffic Id  xstime=Inherited
      settings: SourceProductName=CarMaker4SL
  Traffic_Info : Outport
  wires:
  ObjectId_T00/1 -> Traffic Object T00/1
  Traffic Object T00/1 -> Terminator_T00/1
  Traffic Object T00/2 -> Bus Selector T00/1
  Bus Selector T00/1 -> Mux_T00/1  "<t_0 x>"
  Bus Selector T00/2 -> Mux_T00/2  "<t_0 y>"
  Bus Selector T00/3 -> Mux_T00/3  "<r_zyx z>"
  ObjectId_T01/1 -> Traffic Object T01/1
  Traffic Object T01/1 -> Terminator_T01/1
  Traffic Object T01/2 -> Bus Selector T01/1
  Bus Selector T01/1 -> Mux_T01/1  "<t_0 x>"
  Bus Selector T01/2 -> Mux_T01/2  "<t_0 y>"
  Bus Selector T01/3 -> Mux_T01/3  "<r_zyx z>"
  ObjectId_T02/1 -> Traffic Object T02/1
  Traffic Object T02/1 -> Terminator_T02/1
  Traffic Object T02/2 -> Bus Selector T02/1
  Bus Selector T02/1 -> Mux_T02/1  "<t_0 x>"
  Bus Selector T02/2 -> Mux_T02/2  "<t_0 y>"
  Bus Selector T02/3 -> Mux_T02/3  "<r_zyx z>"
  ObjectId_T03/1 -> Traffic Object T03/1
  Traffic Object T03/1 -> Terminator_T03/1
  Traffic Object T03/2 -> Bus Selector T03/1
  Bus Selector T03/1 -> Mux_T03/1  "<t_0 x>"
  Bus Selector T03/2 -> Mux_T03/2  "<t_0 y>"
  Bus Selector T03/3 -> Mux_T03/3  "<r_zyx z>"
  ObjectId_T04/1 -> Traffic Object T04/1
  Traffic Object T04/1 -> Terminator_T04/1
  Traffic Object T04/2 -> Bus Selector T04/1
  Bus Selector T04/1 -> Mux_T04/1  "<t_0 x>"
  Bus Selector T04/2 -> Mux_T04/2  "<t_0 y>"
  Bus Selector T04/3 -> Mux_T04/3  "<r_zyx z>"
  ObjectId_T05/1 -> Traffic Object T05/1
  Traffic Object T05/1 -> Terminator_T05/1
  Traffic Object T05/2 -> Bus Selector T05/1
  Bus Selector T05/1 -> Mux_T05/1  "<t_0 x>"
  Bus Selector T05/2 -> Mux_T05/2  "<t_0 y>"
  Bus Selector T05/3 -> Mux_T05/3  "<r_zyx z>"
  ObjectId_T06/1 -> Traffic Object T06/1
  Traffic Object T06/1 -> Terminator_T06/1
  Traffic Object T06/2 -> Bus Selector T06/1
  Bus Selector T06/1 -> Mux_T06/1  "<t_0 x>"
  Bus Selector T06/2 -> Mux_T06/2  "<t_0 y>"
  Bus Selector T06/3 -> Mux_T06/3  "<r_zyx z>"
  ObjectId_T07/1 -> Traffic Object T07/1
  Traffic Object T07/1 -> Terminator_T07/1
  Traffic Object T07/2 -> Bus Selector T07/1
  Bus Selector T07/1 -> Mux_T07/1  "<t_0 x>"
  Bus Selector T07/2 -> Mux_T07/2  "<t_0 y>"
  Bus Selector T07/3 -> Mux_T07/3  "<r_zyx z>"
  ObjectId_T08/1 -> Traffic Object T08/1
  Traffic Object T08/1 -> Terminator_T08/1
  Traffic Object T08/2 -> Bus Selector T08/1
  Bus Selector T08/1 -> Mux_T08/1  "<t_0 x>"
  Bus Selector T08/2 -> Mux_T08/2  "<t_0 y>"
  Bus Selector T08/3 -> Mux_T08/3  "<r_zyx z>"
  ObjectId_T09/1 -> Traffic Object T09/1
  Traffic Object T09/1 -> Terminator_T09/1
  Traffic Object T09/2 -> Bus Selector T09/1
  Bus Selector T09/1 -> Mux_T09/1  "<t_0 x>"
  Bus Selector T09/2 -> Mux_T09/2  "<t_0 y>"
  Bus Selector T09/3 -> Mux_T09/3  "<r_zyx z>"
  ObjectId_T10/1 -> Traffic Object T10/1
  Traffic Object T10/1 -> Terminator_T10/1
  Traffic Object T10/2 -> Bus Selector T10/1
  Bus Selector T10/1 -> Mux_T10/1  "<t_0 x>"
  Bus Selector T10/2 -> Mux_T10/2  "<t_0 y>"
  Bus Selector T10/3 -> Mux_T10/3  "<r_zyx z>"
  ObjectId_T11/1 -> Traffic Object T11/1
  Traffic Object T11/1 -> Terminator_T11/1
  Traffic Object T11/2 -> Bus Selector T11/1
  Bus Selector T11/1 -> Mux_T11/1  "<t_0 x>"
  Bus Selector T11/2 -> Mux_T11/2  "<t_0 y>"
  Bus Selector T11/3 -> Mux_T11/3  "<r_zyx z>"
  ObjectId_T12/1 -> Traffic Object T12/1
  Traffic Object T12/1 -> Terminator_T12/1
  Traffic Object T12/2 -> Bus Selector T12/1
  Bus Selector T12/1 -> Mux_T12/1  "<t_0 x>"
  Bus Selector T12/2 -> Mux_T12/2  "<t_0 y>"
  Bus Selector T12/3 -> Mux_T12/3  "<r_zyx z>"
  ObjectId_T13/1 -> Traffic Object T13/1
  Traffic Object T13/1 -> Terminator_T13/1
  Traffic Object T13/2 -> Bus Selector T13/1
  Bus Selector T13/1 -> Mux_T13/1  "<t_0 x>"
  Bus Selector T13/2 -> Mux_T13/2  "<t_0 y>"
  Bus Selector T13/3 -> Mux_T13/3  "<r_zyx z>"
  ObjectId_T14/1 -> Traffic Object T14/1
  Traffic Object T14/1 -> Terminator_T14/1
  Traffic Object T14/2 -> Bus Selector T14/1
  Bus Selector T14/1 -> Mux_T14/1  "<t_0 x>"
  Bus Selector T14/2 -> Mux_T14/2  "<t_0 y>"
  Bus Selector T14/3 -> Mux_T14/3  "<r_zyx z>"
  ObjectId_T15/1 -> Traffic Object T15/1
  Traffic Object T15/1 -> Terminator_T15/1
  Traffic Object T15/2 -> Bus Selector T15/1
  Bus Selector T15/1 -> Mux_T15/1  "<t_0 x>"
  Bus Selector T15/2 -> Mux_T15/2  "<t_0 y>"
  Bus Selector T15/3 -> Mux_T15/3  "<r_zyx z>"
  ObjectId_T16/1 -> Traffic Object T16/1
  Traffic Object T16/1 -> Terminator_T16/1
  Traffic Object T16/2 -> Bus Selector T16/1
  Bus Selector T16/1 -> Mux_T16/1  "<t_0 x>"
  Bus Selector T16/2 -> Mux_T16/2  "<t_0 y>"
  Bus Selector T16/3 -> Mux_T16/3  "<r_zyx z>"
  ObjectId_T17/1 -> Traffic Object T17/1
  Traffic Object T17/1 -> Terminator_T17/1
  Traffic Object T17/2 -> Bus Selector T17/1
  Bus Selector T17/1 -> Mux_T17/1  "<t_0 x>"
  Bus Selector T17/2 -> Mux_T17/2  "<t_0 y>"
  Bus Selector T17/3 -> Mux_T17/3  "<r_zyx z>"
  ObjectId_T18/1 -> Traffic Object T18/1
  Traffic Object T18/1 -> Terminator_T18/1
  Traffic Object T18/2 -> Bus Selector T18/1
  Bus Selector T18/1 -> Mux_T18/1  "<t_0 x>"
  Bus Selector T18/2 -> Mux_T18/2  "<t_0 y>"
  Bus Selector T18/3 -> Mux_T18/3  "<r_zyx z>"
  ObjectId_T19/1 -> Traffic Object T19/1
  Traffic Object T19/1 -> Terminator_T19/1
  Traffic Object T19/2 -> Bus Selector T19/1
  Bus Selector T19/1 -> Mux_T19/1  "<t_0 x>"
  Bus Selector T19/2 -> Mux_T19/2  "<t_0 y>"
  Bus Selector T19/3 -> Mux_T19/3  "<r_zyx z>"
  ObjectId_T20/1 -> Traffic Object T20/1
  Traffic Object T20/1 -> Terminator_T20/1
  Traffic Object T20/2 -> Bus Selector T20/1
  Bus Selector T20/1 -> Mux_T20/1  "<t_0 x>"
  Bus Selector T20/2 -> Mux_T20/2  "<t_0 y>"
  Bus Selector T20/3 -> Mux_T20/3  "<r_zyx z>"
  Mux_T00/1 -> Mux_Traffic_Info_All/1
  Mux_T01/1 -> Mux_Traffic_Info_All/2
  Mux_T02/1 -> Mux_Traffic_Info_All/3
  Mux_T03/1 -> Mux_Traffic_Info_All/4
  Mux_T04/1 -> Mux_Traffic_Info_All/5
  Mux_T05/1 -> Mux_Traffic_Info_All/6
  Mux_T06/1 -> Mux_Traffic_Info_All/7
  Mux_T07/1 -> Mux_Traffic_Info_All/8
  Mux_T08/1 -> Mux_Traffic_Info_All/9
  Mux_T09/1 -> Mux_Traffic_Info_All/10
  Mux_T10/1 -> Mux_Traffic_Info_All/11
  Mux_T11/1 -> Mux_Traffic_Info_All/12
  Mux_T12/1 -> Mux_Traffic_Info_All/13
  Mux_T13/1 -> Mux_Traffic_Info_All/14
  Mux_T14/1 -> Mux_Traffic_Info_All/15
  Mux_T15/1 -> Mux_Traffic_Info_All/16
  Mux_T16/1 -> Mux_Traffic_Info_All/17
  Mux_T17/1 -> Mux_Traffic_Info_All/18
  Mux_T18/1 -> Mux_Traffic_Info_All/19
  Mux_T19/1 -> Mux_Traffic_Info_All/20
  Mux_T20/1 -> Mux_Traffic_Info_All/21
  Mux_Traffic_Info_All/1 -> Traffic_Info/1
